simulink model "motor_driver"  (R2017b)
settings: Solver=ode3  StartTime=0.0  StopTime=0.5  FixedStep=0.0002  RelTol=1e-3
libraries: stellaris_lp_lib x4, simulink x3
settings Model: ExtModeTrigDuration=2  Creator=peselnikmg  LastModifiedBy=Joshua
settings DataIOCC: LimitDataPoints=on  SaveFormat=Array  SignalLoggingSaveFormat=ModelDataLogs
settings OptimizationCC: PassReuseOutputArgsAs=Individual arguments  ExpressionDepthLimit=2147483647  MaxStackSize=64
settings DebuggingCC: ParameterTunabilityLossMsg=error  StateNameClashWarn=warning  SFUnexpectedBacktrackingDiag=warning  SFNoUnconditionalDefaultTransitionDiag=warning  SFExecutionAtInitializationDiag=none
settings HardwareCC: ProdBitPerPointer=32  ProdBitPerSizeT=32  ProdBitPerPtrDiffT=32  ProdLargestAtomicInteger=Long  ProdLargestAtomicFloat=Double  ProdWordSize=32  ProdHWDeviceType=ARM Compatible->ARM Cortex
settings ModelReferenceCC: PropagateSignalLabelsOutOfModel=off
settings SFSimCC: MATLABDynamicMemAlloc=off
settings RTWCC: SystemTargetFile=ert.tlc  HardwareBoard=Tiva TM4C123G Launchpad  TLCOptions=-aInlineSetEventsForThisBaseRateFcn=TLC_FALSE -aSuppressMultiTaskScheduler=TLC_FALSE -aRateBasedStepFcn=1  TemplateMakefile=ert_default_tmf  GenerateReport=on  RTWVerbose=off  Toolchain=Texas Instruments Code Composer Studio (Tiva)  IncludeHyperlinkInReport=on  LaunchReport=on  GenerateTraceInfo=on  GenerateTraceReport=on  GenerateTraceReportSl=on  GenerateTraceReportSf=on  GenerateTraceReportEml=on
settings CodeAppCC: ForceParamTrailComments=on  IgnoreCustomStorageClasses=off  OperatorAnnotations=on  SimulinkDataObjDesc=on  SFDataObjDesc=on  MATLABFcnDesc=on  CustomSymbolStrType=$N$R$M  InsertBlockDesc=on  StateflowObjectComments=on  MATLABSourceComments=on  InternalIdentifier=Classic
settings ConfigComp: CovMetricSettings=dw  CovHtmlReporting=on  CovSaveCumulativeToWorkspaceVar=on  CovSaveSingleToWorkspaceVar=on  CovExternalEMLEnable=off
settings SimscapeCC: SimscapeNormalizeSystem=off

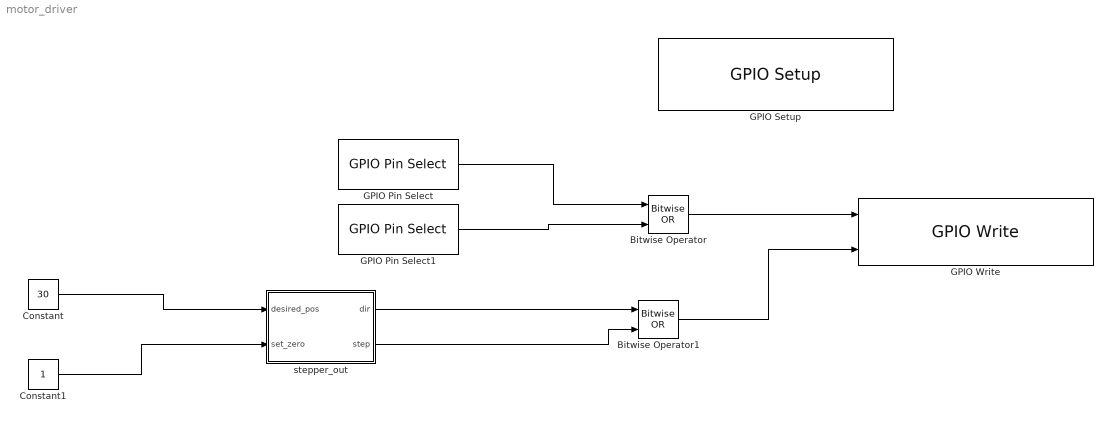
== system motor_driver ==
  Bitwise Operator : simulink/Logic and Bit Operations/Bitwise Operator  logicop=OR  UseBitMask=off  NumInputPorts=2  BitMask=bin2dec('11011001')  BitMaskRealWorld=Stored Integer
  Bitwise Operator1 : simulink/Logic and Bit Operations/Bitwise Operator  logicop=OR  UseBitMask=off  NumInputPorts=2  BitMask=bin2dec('11011001')  BitMaskRealWorld=Stored Integer
  Constant : Constant  Value=30
  Constant1 : Constant
  GPIO Pin Select : stellaris_lp_lib/GPIO/GPIO Pin Select  GPIO_PIN_X=GPIO_PIN_2
      settings: SourceProductName=Run on Stellaris LaunchPad
  GPIO Pin Select1 : stellaris_lp_lib/GPIO/GPIO Pin Select  GPIO_PIN_X=GPIO_PIN_3
      settings: SourceProductName=Run on Stellaris LaunchPad
  GPIO Setup : stellaris_lp_lib/GPIO/GPIO Setup  GPIO_PORTX_BASE=GPIO_PORTF_BASE  PinsOutput_0=Unused  PinsOutput_1=Unused  PinsOutput_2=Output  PinsOutput_3=Output  PinsOutput_4=Unused  PinsOutput_5=Unused  PinsOutput_6=Unused  PinsOutput_7=Unused
      settings: SourceProductName=Run on Stellaris LaunchPad
  GPIO Write : stellaris_lp_lib/GPIO/GPIO Write  GPIO_PORTX_BASE=GPIO_PORTF_BASE  SampleTime=-1
      settings: SourceProductName=Run on Stellaris LaunchPad
  stepper_out : Subsystem
  wires:
  Bitwise Operator/1 -> GPIO Write/1
  GPIO Pin Select/1 -> Bitwise Operator/1
  GPIO Pin Select1/1 -> Bitwise Operator/2
  stepper_out/1(dir) -> Bitwise Operator1/1
  stepper_out/2(step) -> Bitwise Operator1/2
  Bitwise Operator1/1 -> GPIO Write/2
  Constant/1 -> stepper_out/1(desired_pos)
  Constant1/1 -> stepper_out/2(set_zero)

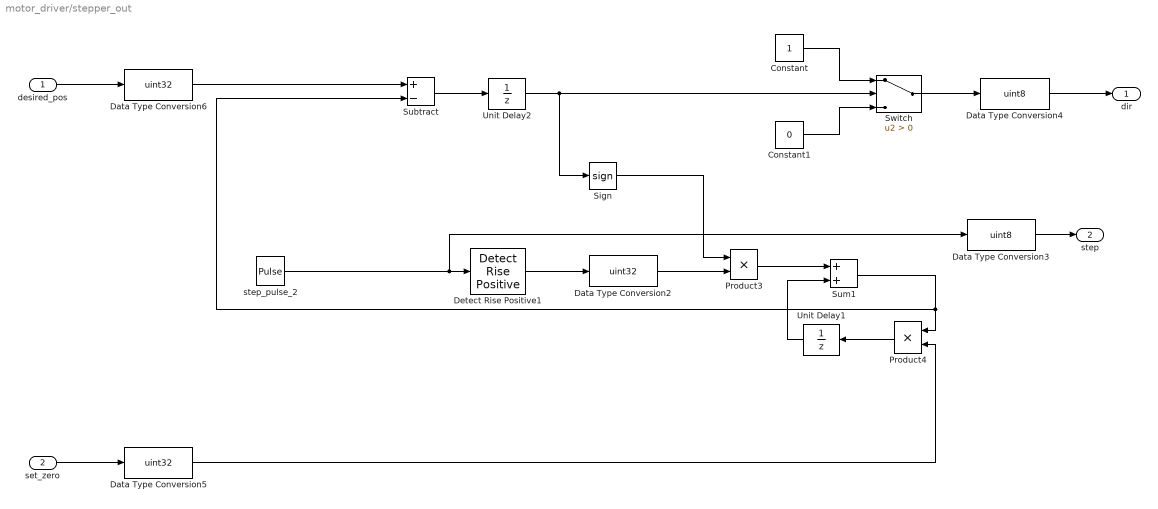
== system motor_driver/stepper_out ==
  desired_pos : Inport
  set_zero : Inport  Port=2
  Constant : Constant
  Constant1 : Constant  Value=0
  Data Type Conversion2 : DataTypeConversion  OutDataTypeStr=uint32
  Data Type Conversion3 : DataTypeConversion  OutDataTypeStr=uint8
  Data Type Conversion4 : DataTypeConversion  OutDataTypeStr=uint8
  Data Type Conversion5 : DataTypeConversion  OutDataTypeStr=uint32
  Data Type Conversion6 : DataTypeConversion  OutDataTypeStr=uint32
  Detect Rise Positive1 : simulink/Logic and Bit Operations/Detect Rise Positive  vinit=0  OutDataTypeStr=boolean
  Product3 : Product  OutDataTypeStr=uint32
  Product4 : Product  OutDataTypeStr=uint32
  Sign : Signum
  Subtract : Sum  Inputs=+-  AccumDataTypeStr=uint32
  Sum1 : Sum  AccumDataTypeStr=uint32  OutDataTypeStr=uint32  SaturateOnIntegerOverflow=on
  Switch : Switch  Criteria=u2 > Threshold  OutDataTypeStr=uint8
  Unit Delay1 : UnitDelay  SampleTime=-1
  Unit Delay2 : UnitDelay  SampleTime=-1
  step_pulse_2 : DiscretePulseGenerator  PulseType=Time based  Amplitude=2^2  Period=0.002  PulseWidth=50
  dir : Outport
  step : Outport  Port=2
  wires:
  Detect Rise Positive1/1 -> Data Type Conversion2/1
  Data Type Conversion2/1 -> Product3/2
  Product3/1 -> Sum1/1
  Unit Delay1/1 -> Sum1/2
  Product4/1 -> Unit Delay1/1
  Sum1/1 -> Subtract/2, Product4/1
  set_zero/1 -> Data Type Conversion5/1
  desired_pos/1 -> Data Type Conversion6/1
  Subtract/1 -> Unit Delay2/1
  Sign/1 -> Product3/1
  Switch/1 -> Data Type Conversion4/1
  step_pulse_2/1 -> Data Type Conversion3/1, Detect Rise Positive1/1
  Constant1/1 -> Switch/3
  Constant/1 -> Switch/1
  Data Type Conversion4/1 -> dir/1
  Data Type Conversion3/1 -> step/1
  Data Type Conversion5/1 -> Product4/2
  Data Type Conversion6/1 -> Subtract/1
  Unit Delay2/1 -> Switch/2, Sign/1
